simulink model "Trajectory"  (R2024b)
settings: Solver=VariableStepAuto  StartTime=0.0  StopTime=10.0  RelTol=1e-3
libraries: slpidlib x10
(part 2 of 2)

== matlab function Trajectory/Trajectory Controller/Lateral Controller/Lateral Linerasation Matrices ==
  data: u input; x_dot_lat output; x_lat input; u_lat input
function x_dot_lat = Lat_linear(u, x_lat, u_lat)
% Author:
%   Hanchen Li (hl3422@ic.ac.uk)
%
% Inputs:
%   x_lat     - [v, p, r, phi, psi]
%   v         - Lateral velocity (m/s)
%   p         - Roll rate (rad/s)
%   r         - Yaw rate (rad/s)
%   phi       - Euler roll angle (rad)
%   psi       - Euler yaw angle (rad)
%
%   u_lat      - [theta_diff, theta_1c, delta_R]
%   theta_diff - Rotor collective difference (rad)
%   theta_1c   - Lateral cyclic (rad)
%   delta_R    - Rudder deflection (rad)
%
%   u         - Forward velocity (m/s)
%
% Outputs:
%   x_dot_lat     - [v_dot, p_dot, r_dot, phi_dot, psi_dot]

%% 0 Extract Parameters
% v          = x_lat(1);
% p          = x_lat(2);
% r          = x_lat(3);
% phi        = x_lat(4);
% psi        = x_lat(5);

% theta_diff = u_lat(1);
% theta_1c   = u_lat(2);
% delta_R    = u_lat(3);

%% 1 Initial parameters
U = [0; 20; 40; 60; 72.0222222]; % 5 break-points

A_lat_all = cat(3,...
[-0.00723803596901745	0.766629187912504	0	9.80664998365558	0;
-0.0220588605968897	2.33772683898305	0	0	0;
-0.00849763594524569	0.895100650677353	0	0	0;
0	1	-3.37129866355175e-20	0	0;
0	0	1	0	0], ...
[-0.0287466714637974	-0.899953672094944	-20.0000000000000	9.80490709913392	0;
0.0630234288050327	-42.8490378164358	0	0	0;
0.0165241972871400	-16.4084615444215	0	0	0;
0	1	-0.00133938338078559	0	0;
0	0	0.999824069502805	0	0],...
[-0.0614472963440804	-0.794593411243688	-40.0000000000000	9.80045162928003	0;
0.0921179719871219	-44.7576558257473	0	0	0;
0.0201395907071134	-17.1415154344742	0	0	0;
0	1	-0.0258480649251392	0	0;
0	0	1.00003604213456	0	0],...
[-0.0939985407377719	-0.553352915029781	-60.0000000000001	9.80470081610160	0;
0.137754655670817	-44.4145547554134	0	0	0;
0.0300442349300036	-17.0089253466231	0	0	0;
0	1	-0.00745253368129878	0	0;
0	0	0.999856788437422	0	0],...
[-0.113487618299962	-0.474169631164562	-72.0222222000000	9.80530163216295	0;
0.186394218922800	-44.6707815075849	0	0	0;
0.0441186726466513	-17.1062286441804	0	0	0;
0	1	0.00525336319929938	0	0;
0	0	0.999890107270042	0	0]);

B_lat_all = cat(3,...
[3.23169927067643e-19	-5.17979000748556	0;
39.4348460540525	-15.7950340421649	0;
20.0367522163849	-6.04781748357008	0;
0	0	0;
0	0	0],...
[4.31696975593948	5.82238189586901	-0.609135989935172;
-23.0678427461869	436.624054048141	-0.483823191299985;
-8.82007681597619	167.170048738641	-0.337234009306154;
0	0	0;
0	0	0],...
[7.22875419412211	5.19111587446400	-2.42771590191537;
-57.6629781774963	465.505315642842	-1.92828083489087;
-22.1058230727191	178.212733876920	-1.34404858781424;
0	0	0;
0	0	0],...
[8.40285260125251	3.79379187492618	-5.46236077930973;
-25.0260057506118	456.385397516595	-4.33863187850467;
-9.61025631477467	174.689455049333	-3.02410932258211;
0	0	0;
0	0	0],...
[8.61969410886620	3.36925382550327	-7.87065569844800;
-19.7749208552367	470.879026333778	-6.25148705800775;
-7.60984268371909	180.231587049336	-4.35740593383498;
0	0	0;
0	0	0]);

%% 2 Vectorised interpolation
method = 'pchip';

A_lat =  squeeze( interp1(U, permute(A_lat_all,[3 1 2]), u, method, 'extrap') );
B_lat =  squeeze( interp1(U, permute(B_lat_all,[3 1 2]), u, method, 'extrap') );

%% 3 Output
x_dot_lat = A_lat * x_lat + B_lat * u_lat;

end

== matlab function Trajectory/Trajectory Controller/Lateral Controller/Blend Factor ==
  data: blend output; u input
function blend = Blend_yaw(u)
% Author:
%   Hanchen Li (hl3422@ic.ac.uk)
%
% Inputs:
%   u         - Forward velocity (m/s)
%
% Outputs:
%   blend     - blend factor

if abs(u) < 1e-4

    blend = 0;

elseif abs(u) < 90.3

    blend = u / (90.3 / 0.8);

else

    blend = 0.8;

end

end

== matlab function Trajectory/Trajectory Controller/Lateral Controller/Heading Hold/Wrap Angle ==
  data: e_chi output; e input
function e_chi = Wrap_Pi(e)
% Author:
%   Hanchen Li (hl3422@ic.ac.uk)
%
% Inputs:
%   chi
%
% Outputs:
%   e_chi

e_chi = mod(chi + pi, 2 * pi) - pi;

end

== matlab function Trajectory/Trajectory Controller/Longitudinal Controller/Collective Pitch Trim Condition ==
  data: u input; theta_UR output; theta_LR output
function [theta_UR, theta_LR] = Trim_collective(u)
% Author:
%   Hanchen Li (hl3422@ic.ac.uk)
%
% Inputs:
%   u         - Forward velocity (m/s)
%
% Outputs:
%   theta_LR  - Lower rotor collective (rad)
%   theta_UR  - Upper rotor collective (rad)

% Trim Point
v_F_t = 72.0222222; % 140 knots = 72.0222222 m/s

% Forward Flight
% from 0 to 84.7 m/s
v_F = [0, 15, 30, 45, 60, v_F_t, 90.3];

% Linearization Point
% Hover
theta_LR_H_4 = 0.2198;
theta_UR_H_4 = 0.2661;

% Trim Point
theta_LR_t_4 = 0.1717;
theta_UR_t_4 = 0.1602;

% Forward Flight
theta_LR_F_4 = [theta_LR_H_4, 0.1900, 0.1770, 0.1657, 0.1665, theta_LR_t_4, 0.1928];
theta_UR_F_4 = [theta_UR_H_4, 0.1113, 0.1078, 0.1274, 0.1427, theta_UR_t_4, 0.1909];

v_F_fine = linspace(min(v_F), max(v_F), 500);
theta_LR_F_4_interp = interp1(v_F, theta_LR_F_4, v_F_fine, 'pchip');
theta_UR_F_4_interp = interp1(v_F, theta_UR_F_4, v_F_fine, 'pchip');

[~, idx]   = min(abs(v_F_fine - u));

theta_LR = theta_LR_F_4_interp(idx);
theta_UR = theta_UR_F_4_interp(idx);

end

== matlab function Trajectory/Plot Trajectory ==
  data: x_E_ref input; y_E_ref input; z_E_ref input; x_E input; y_E input; z_E input
function plot3D(x_E_ref, y_E_ref, z_E_ref, x_E, y_E, z_E)
% Author:
%   Hanchen Li (hl3422@ic.ac.uk)
%
% Inputs:
%   x_E_ref   - Distance in the Earth x-direction (m/s)
%   x_E_ref   - Distance in the Earth x-direction (m/s)
%   x_E_ref   - Distance in the Earth x-direction (m/s)
%   x_E       - Distance in the Earth x-direction (m/s)
%   x_E       - Distance in the Earth x-direction (m/s)
%   x_E       - Distance in the Earth x-direction (m/s)
%
% Outputs:
%   Real time 3D trajectory plot

% Persistent line objects for plotting
persistent refLine actLine firstRun

% Initialization (on first call)
if isempty(firstRun)
    
    figure(1); clf;
    refLine = animatedline('Color', [0/255 0/255 128/255], 'LineStyle', '--', 'LineWidth', 1.5, 'DisplayName', 'Reference');
    actLine = animatedline('Color', [220/255 20/255 60/255], 'LineStyle', '-',  'LineWidth', 1.5, 'DisplayName', 'Actual');
    xlabel('x_E'); ylabel('y_E'); zlabel('z_E');
    title('HALO 3-D trajectory plot.');
    grid on;
    view(3);
    legend show;
    axis equal;
    hold on;
    firstRun = true;
end

% Add new points
addpoints(refLine, x_ref, y_ref, z_ref);
addpoints(actLine, x, y, z);
    
% Update plot
drawnow limitrate;

end

== matlab function Trajectory/Navigation Equation ==
  data: x_dot_E output; y_dot_E output; z_dot_E output; state input
function [x_dot_E, y_dot_E, z_dot_E] = Navigation(state)
% Author:
%   Hanchen Li (hl3422@ic.ac.uk)
%
% Inputs:
%   state     - [u, v, w, p, q, r, phi, theta, psi]
%   u         - Forward velocity (m/s)
%   v         - Lateral velocity (m/s)
%   w         - Vertical velocity (m/s)
%   p         - Roll rate (rad/s)
%   q         - Pitch rate (rad/s)
%   r         - Yaw rate (rad/s)
%   phi       - Euler roll angle (rad)
%   theta     - Euler pitch angle (rad)
%   psi       - Euler yaw angle (rad)
%
% Outputs:
%   x_dot_E   - Velocity in the Earth x-direction (m/s)
%   y_dot_E   - Velocity in the Earth y-direction (m/s)
%   z_dot_E   - Velocity in the Earth z-direction (m/s)

%% 0 Basic Parameters

% 0.1 Extract parameters
% state - [u, v, w, p, q, r, phi, theta, psi]
u = state(1);
v = state(2);
w = state(3);
p = state(4);
q = state(5);
r = state(6);
phi = state(7);
theta = state(8);
psi = state(9);

% 0.2 Compute trigonometric values
cphi = cos(phi);
sphi = sin(phi);
ctheta = cos(theta);
stheta = sin(theta);
cpsi = cos(psi);
spsi = sin(psi);

% 0.3 Transformation matrix from body to inertial frame
T = [...
     ctheta * cpsi, sphi * stheta * cpsi - cphi * spsi, cphi * stheta * cpsi + sphi * spsi;
     ctheta * spsi, sphi * stheta * spsi + cphi * cpsi, cphi * stheta * spsi - sphi * cpsi;
     -stheta      , sphi * ctheta                     , cphi * ctheta];

%% 1 Calculation
% 1.1 Body velocity vector
V_body = [u; v; w];

% 1.2 Compute inertial velocity
V_inertial = T * V_body;

% 1.3 Output
x_dot_E = V_inertial(1);
y_dot_E = V_inertial(2);
z_dot_E = V_inertial(3);

end

== matlab function Trajectory/Trajectory Controller/Combine State ==
  data: x output; x_lon input; x_lat input
function x = Combine_State(x_lon, x_lat)
% Author:
%   Hanchen Li (hl3422@ic.ac.uk)
%
% Inputs:
%   x_lon     - [u, w, q, theta]
%   u         - Forward velocity (m/s)
%   w         - Vertical velocity (m/s)
%   q         - Pitch rate (rad/s)
%   theta     - Euler pitch angle (rad)
%
%   x_lat     - [v, p, r, phi, psi]
%   v         - Lateral velocity (m/s)
%   p         - Roll rate (rad/s)
%   r         - Yaw rate (rad/s)
%   phi       - Euler roll angle (rad)
%   psi       - Euler yaw angle (rad)
%
% Outputs:
%   x         - [u, v, w, p, q, r, phi, theta, psi]
%   u         - Forward velocity (m/s)
%   v         - Lateral velocity (m/s)
%   w         - Vertical velocity (m/s)
%   p         - Roll rate (rad/s)
%   q         - Pitch rate (rad/s)
%   r         - Yaw rate (rad/s)
%   phi       - Euler roll angle (rad)
%   theta     - Euler pitch angle (rad)
%   psi       - Euler yaw angle (rad)

%% 0 Extract Parameters

% x_lon - [u, w, q, theta]
u     = x_lon(1);
w     = x_lon(2);
q     = x_lon(3);
theta = x_lon(4);

% x_lat - [v, p, r, phi, psi]
v     = x_lat(1);
p     = x_lat(2);
r     = x_lat(3);
phi   = x_lat(4);
psi   = x_lat(5);

%% 1 Combination

x = [u, v, w, p, q, r, phi, theta, psi];

end

== matlab function Trajectory/Trajectory Controller/Combine Control ==
  data: u output; u_lon input; u_lat input
function u = Combine_Control(u_lon, u_lat)
% Author:
%   Hanchen Li (hl3422@ic.ac.uk)
%
% Inputs:
%   u_lon      - [theta_0, theta_1s, delta_E]
%   theta_0    - Average rotor collective (rad)
%   theta_1s   - Longitudinal cyclic (rad)
%   delta_E    - Elevator deflection (rad)
%
%   u_lat      - [theta_diff, theta_1c, delta_R]
%   theta_diff - Rotor collective difference (rad)
%   theta_1c   - Lateral cyclic (rad)
%   delta_R    - Rudder deflection (rad)
%
% Outputs:
%   u          - [theta_LR, theta_UR, theta_1s, theta_1c, delta_E, delta_R]
%   theta_LR   - Lower rotor collective (rad)
%   theta_UR   - Upper rotor collective (rad)
%   theta_1s   - Longitudinal cyclic (rad)
%   theta_1c   - Lateral cyclic (rad)
%   delta_E    - Elevator deflection (rad)
%   delta_R    - Rudder deflection (rad)

%% 0 Extract Parameters

% u_lon - [theta_0, theta_1s, delta_E]
theta_0    = u_lon(1);
theta_1s   = u_lon(2);
delta_E    = u_lon(3);

% u_lat - [theta_diff, theta_1c, delta_R]
theta_diff = u_lat(1);
theta_1c   = u_lat(2);
delta_R    = u_lat(3);

%% 1 Combination

theta_LR = theta_0 - theta_diff / 2;

theta_UR = theta_0 + theta_diff / 2;

u = [theta_LR, theta_UR, theta_1s, theta_1c, delta_E, delta_R];

end

== matlab function Trajectory/Trajectory Controller/Combine State Derivatives ==
  data: x_dot output; x_dot_lon input; x_dot_lat input
function x_dot = Combine_State(x_dot_lon, x_dot_lat)
% Author:
%   Hanchen Li (hl3422@ic.ac.uk)
%
% Inputs:
%   x_lon     - [u, w, q, theta]
%   u         - Forward velocity (m/s)
%   w         - Vertical velocity (m/s)
%   q         - Pitch rate (rad/s)
%   theta     - Euler pitch angle (rad)
%
%   x_lat     - [v, p, r, phi, psi]
%   v         - Lateral velocity (m/s)
%   p         - Roll rate (rad/s)
%   r         - Yaw rate (rad/s)
%   phi       - Euler roll angle (rad)
%   psi       - Euler yaw angle (rad)
%
% Outputs:
%   x         - [u, v, w, p, q, r, phi, theta, psi]
%   u         - Forward velocity (m/s)
%   v         - Lateral velocity (m/s)
%   w         - Vertical velocity (m/s)
%   p         - Roll rate (rad/s)
%   q         - Pitch rate (rad/s)
%   r         - Yaw rate (rad/s)
%   phi       - Euler roll angle (rad)
%   theta     - Euler pitch angle (rad)
%   psi       - Euler yaw angle (rad)

%% 0 Extract Parameters

% x_lon - [u, w, q, theta]
u_dot     = x_dot_lon(1);
w_dot     = x_dot_lon(2);
q_dot     = x_dot_lon(3);
theta_dot = x_dot_lon(4);

% x_lat - [v, p, r, phi, psi]
v_dot     = x_dot_lat(1);
p_dot     = x_dot_lat(2);
r_dot     = x_dot_lat(3);
phi_dot   = x_dot_lat(4);
psi_dot   = x_dot_lat(5);

%% 1 Combination

x_dot = [u_dot, v_dot, w_dot, p_dot, q_dot, r_dot, phi_dot, theta_dot, psi_dot];

end

== matlab function Trajectory/Trajectory Controller/Longitudinal Controller/Blend Factor ==
  data: blend output; x_lon input
function blend = Blend_pitch(x_lon)
% Author:
%   Hanchen Li (hl3422@ic.ac.uk)
%
% Inputs:
%   x_lon     - [u, w, q, theta]
%   u         - Forward velocity (m/s)
%   w         - Vertical velocity (m/s)
%   q         - Pitch rate (rad/s)
%   theta     - Euler pitch angle (rad)
%
% Outputs:
%   blend     - blend factor

%% 0 Extract Parameters

u     = x_lon(1);

%% 1 Decide blend factor

if abs(u) < 1e-4

    blend = 0;

elseif abs(u) < 90.3

    blend = u / (90.3 / 0.8);

else

    blend = 0.8;

end

end

== matlab function Trajectory/Trajectory Controller/Longitudinal Controller/Longitudinal Linerasation Matrices ==
  data: x_dot_lon output; x_lon input; u_lon input
function x_dot_lon = Lon_linear(x_lon, u_lon)
% Author:
%   Hanchen Li (hl3422@ic.ac.uk)
%
% Inputs:
%   x_lon     - [u, w, q, theta]
%   u         - Forward velocity (m/s)
%   w         - Vertical velocity (m/s)
%   q         - Pitch rate (rad/s)
%   theta     - Euler pitch angle (rad)
%
%   u_lon     - [theta_0, theta_1s, delta_E]
%   theta_0   - Average rotor collective (rad)
%   theta_1s  - Longitudinal cyclic (rad)
%   delta_E   - Elevator deflection (rad)
%
% Outputs:
%   x_dot_lon - [u_dot, w_dot, q_dot, theta_dot]

%% 0 Extract Parameters
u     = x_lon(1);
% w     = x_lon(2);
% q     = x_lon(3);
% theta = x_lon(4);

% theta_0 = u_lon(1);
% theta_1s = u_lon(2);
% delta_E = u_lon(3);

%% 1 Initial parameters
U = [0; 20; 40; 60; 72.0222222]; % 5 break-points

A_lon_all = cat(3,...
[-0.00723802383207751	-1.35323092947785e-20	-0.766629187912504	-9.80664998365558;
-3.64153152077051e-10	-0.626783991819480	0	0;
0.000872483038786669	1.53518643043251e-21	0.0942177477514433	0;
0	0	1	0],...
[-0.0112549858980772	0.0371668055628924	-1.18927896465665	-9.80422222650819;
-0.133476123611587	-1.29584894245305	20.8981012783838	-0.0361550902372443;
0.0229512851532743	0.0212311520956117	-1.57834195971935	0;
0	0	0.999823172370649	0],...
[-0.00894644618554263	0.0320555490226915	-1.19654303458228	-9.78886874671681;
0.0177938328871363	-2.75625714952099	41.9669994347238	0.0565348232672847;
0.00544480361520019	0.0390031290231026	-1.68547625422026	0;
0	0	0.999701937133157	0],...
[-0.00115522776185373	0.0138477446845475	-1.25249222634898	-9.78189512322418;
0.129681745697496	-2.84658770249635	62.0992998719228	-0.370385725787514;
-6.84962619262734e-05	0.0554454638454316	-1.71412794300992	0;
0	0	0.999829013944947	0],...
[0.00198907487199834	0.00124807180451603	-1.31545814391634	-9.77936080280246;
0.208959151679622	-2.91377790533787	74.4525040940847	-0.690902155824347;
-0.00261903529268842	0.0663122914709030	-1.76288467057787	0;
0	0	0.999876306745786	0]);

B_lon_all = cat(3,...
[-2.41065865317012e-18	-5.17979000748556	0;
-111.654787649114	0	0;
2.95095583193773e-19	0.636589574236795	0;
0	0	0],...
[3.61243491647048	-7.51807669482774	0.00519991275444581;
-211.546063860615	-28.3860279697912	-0.718873847311841;
-3.72624202744466	-15.9950728844985	-0.301829974738856;
0	0	0],...
[-2.10906781602821	-8.34051477693776	-0.000966485101117076;
-228.851268194816	-60.5903363544424	-2.65783402805475;
-7.49489399091787	-17.9234263896394	-1.11495618916578;
0	0	0],...
[-6.26132311908841	-9.73615029140097	0;
-245.122010910137	-92.4433695878246	-6.00187247789208;
-13.3651657046107	-20.4991398778183	-2.51787921575724;
0	0	0],...
[-9.36734534820370	-11.2809889940346	0;
-257.948569477389	-112.985439522211	-8.64803218389554;
-16.7725921688728	-22.1441400308729	-3.62798452869815;
0	0	0]);

%% 2 Vectorised interpolation
method = 'pchip';

A_lon =  squeeze( interp1(U, permute(A_lon_all,[3 1 2]), u, method, 'extrap') );
B_lon =  squeeze( interp1(U, permute(B_lon_all,[3 1 2]), u, method, 'extrap') );

%% 3 Output
x_dot_lon = A_lon * x_lon + B_lon * u_lon;

end

== matlab function Trajectory/Trajectory Controller/Longitudinal Controller/Transfer to Array ==
  data: delta_E input; u_lon output; theta_1s input; theta_0 input
function u_lon = u_lon_form(delta_E, theta_1s, theta_0)
% Author:
%   Hanchen Li (hl3422@ic.ac.uk)
%
% Inputs:
%   theta_0   - Average rotor collective (rad)
%   theta_1s  - Longitudinal cyclic (rad)
%   delta_E   - Elevator deflection (rad)
%
% Outputs:
%   u_lon     - [theta_0, theta_1s, delta_E]

u_lon = [theta_0, theta_1s, delta_E];

end

== matlab function Trajectory/Trajectory Controller/Lateral Controller/Lateral State Decomposition ==
  data: r output; phi output; p output; x_lat input
function [r, phi, p] = Lat_linear_decomp(x_lat)
% Author:
%   Hanchen Li (hl3422@ic.ac.uk)
%
% Inputs:
%   x_lat     - [v, p, r, phi, psi]
%
% Outputs:
%   v         - Lateral velocity (m/s)
%   p         - Roll rate (rad/s)
%   r         - Yaw rate (rad/s)
%   phi       - Euler roll angle (rad)
%   psi       - Euler yaw angle (rad)

%% 0 Extract Parameters
p          = x_lat(2);
r          = x_lat(3);
phi        = x_lat(4);


end

== matlab function Trajectory/Trajectory Controller/Longitudinal Controller/Longitudinal State Decomposition ==
  data: q output; w output; x_lon input; theta output; u output
function [q, w, theta, u] = Lon_linear_decomp(x_lon)
% Author:
%   Hanchen Li (hl3422@ic.ac.uk)
%
% Inputs:
%   x_lon     - [u, w, q, theta]
%
% Outputs:
%   w         - Vertical velocity (m/s)
%   q         - Pitch rate (rad/s)
%   theta     - Euler pitch angle (rad)
%   u         - Forward velocity (m/s)

u     = x_lon(1);
w     = x_lon(2);
q     = x_lon(3);
theta = x_lon(4);

end
